simulink model "testing2"  (R2013a)
settings: Solver=ode45  StartTime=0.0  StopTime=30  RelTol=1e-3
settings Model: Creator=z  LastModifiedBy=z

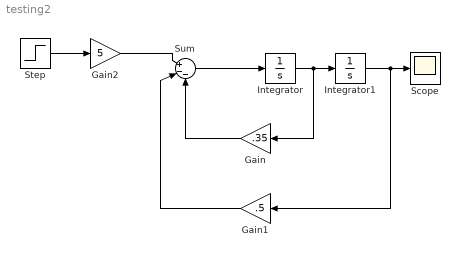
== system testing2 ==
  Gain : Gain  Gain=.35
  Gain1 : Gain  Gain=.5
  Gain2 : Gain  Gain=5
  Integrator : Integrator
  Integrator1 : Integrator
  Scope : Scope
  Step : Step  Time=0  SampleTime=0
  Sum : Sum  Inputs=|+--
  wires:
  Sum/1 -> Integrator/1
  Integrator/1 -> Gain/1, Integrator1/1
  Gain1/1 -> Sum/2
  Integrator1/1 -> Gain1/1, Scope/1
  Gain/1 -> Sum/3
  Step/1 -> Gain2/1
  Gain2/1 -> Sum/1
